simulink model "Robustness"  (R2022a)
settings: Solver=VariableStepAuto  StartTime=0.0  StopTime=10.0  RelTol=1e-3
InitFcn:
  | % NOTE: If using VoltPAQ-X1, make sure both Gain switches are set to 3.
  | K_AMP = 3;
  | % Maximum Output Voltage (V): YAW limited to 15 V. PITCH limited to 24 V.
  | VMAX_AMP_P = 24;
  | VMAX_AMP_Y = 15;
  | % Initial Angle of Pitch (rad)
  | theta_0 = -40.5*pi/180;
  | 
  | g = 9.81;
  | 
  | % Pitch and Yaw Motor Armature Resistance (Ohm)
  | R_m_p = 0.83;
  | R_m_y = 1.60;
  | 
  | % Pitch and Yaw Motor Current-Torque Constant (N.m/A)
  | K_t_p = 0.0182;
  | K_t_y = 0.0109;
  | 
  | % Pitch and Yaw Motor Voltage-Torque Constant (N.m/V)
  | K_yp = K_t_p / R_m_p;
  | K_py = K_t_y / R_m_y;
  | 
  | % Pitch and Yaw Viscous Damping Constant (N.m.s/rad)
  | B_p = 0.8;  % tuned while running simulation and experiment in parallel
  | B_y = 0.318; % identified as described in manual
  | 
  | % Mass of the Helicopter (kg)
  | m_heli = 1.3872;
  | 
  | % Mass of the Helicopter with Yoke (kg)
  | m_heli_case = 1.421;
  | 
  | % Distance from Pitch Pivot to Pitch/Front Motor and Yaw/Back Motor(m)
  | r_p = 7.75*0.0254;
  | r_y = (6+5/8)*0.0254;
  | 
  | % Pitch and Yaw Propeller Force-Thrust Constant found Experimentally (N/V)
  | K_f_p = 5*0.2074;
  | K_f_y = 3*0.1426;
  | 
  | % Pitch and Yaw Propeller Torque-Thrust Constant found Experimentally (N.m/V)
  | K_pp = K_f_p * r_p;
  | K_yy = K_f_y * r_y;
  | 
  | % Mass of Pitch/Front Motor and Yaw/Back Motor (kg)
  | m_motor_p = 0.292;
  | m_motor_y = 0.128;
  | 
  | % Mass of Pitch/Front and Yaw/Back Guard + Propeller(kg)
  | m_shield = 0.143 + 0.024;
  | 
  | % Total Mass of Pitch and Yaw Motor/Shield Assemblies (kg)
  | m_props = ( m_motor_p + m_motor_y + 2 * m_shield );
  | 
  | % Mass of Helicopter Body moving about Pitch Axis (kg)
  | m_body_p = m_heli - m_props;
  | 
  | % Mass of Helicopter Body moving about Yaw Axis (kg)
  | m_body_y = m_heli_case - m_props;
  | 
  | % Mass of Metal Shaft Moving about Yaw Axis (kg)
  | m_shaft = 0.151;
  | 
  | % Total Length of Helicopter Body (m)
  | L_body = 19*0.0254;
  | 
  | % Helicopter Center of Mass from Pivot along Pitch Axis (m)
  | l_cm = ( (m_motor_p + m_shield ) * r_p +  (m_motor_y + m_shield ) * r_y ) / ( m_props ) ;
  | 
  | % Length of Metal Shaft Moving about Yaw Axis through slip ring (m)
  | L_shaft = 11 * 0.0254;
  | 
  | % Pitch and Yaw Motor Rotor Moment of Inertia (kg.m^2)
  | J_m_p = 1.91e-6; %1.7070e-5;
  | J_m_y = 1.374e-4; %1.4471e-5;
  | 
  | % Moment of Inertia of Helicopter Body about its CM (kg.m^2)
  | J_body_p = m_body_p * L_body^2 / 12;
  | J_body_y = m_body_y * L_body^2 / 12;
  | 
  | % Moment of Inertia of Metal Shaft about Yaw Axis (kg.m^2)
  | J_shaft = m_shaft * L_shaft^2 / 3; %;0.0851;
  | 
  | % Moment of Inertia of Pitch Motor + Guard Assembly about Pivot (kg.m^2)
  | J_p = ( m_motor_p + m_shield ) * r_p^2;
  | 
  | % Moment of Inertia of Yaw Motor + Guard Assembly about Pivot (kg.m^2)
  | J_y = ( m_motor_y + m_shield ) * r_y^2;
  | 
  | % Equivalent Moment of Inertia about Pitch and Yaw Axis (kg.m^2)
  | J_eq_p = J_m_p + J_body_p + J_p + J_y;
  | J_eq_y = J_m_y + J_body_y + J_p + J_y + J_shaft;
  | 
  | 
  | %BESSEL wn=4
  | Kbes=[     68.5119  -25.1203    5.3421   -3.6881
  |    63.1652  188.4894    0.7783   19.4789];
  | 
  | xd=-20;
settings Model: Creator=rezan  LastModifiedBy=rezan

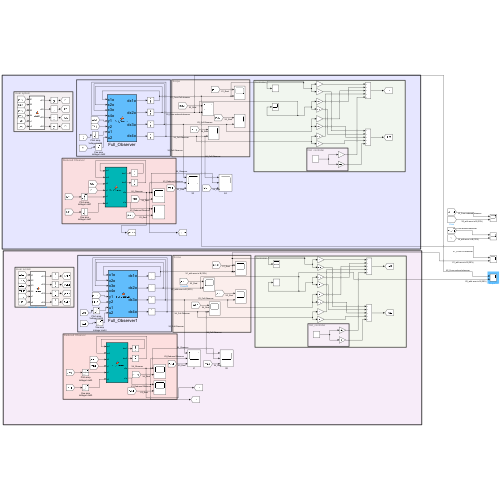
[thumbnail: Simulink's stored preview of the top-level diagram]
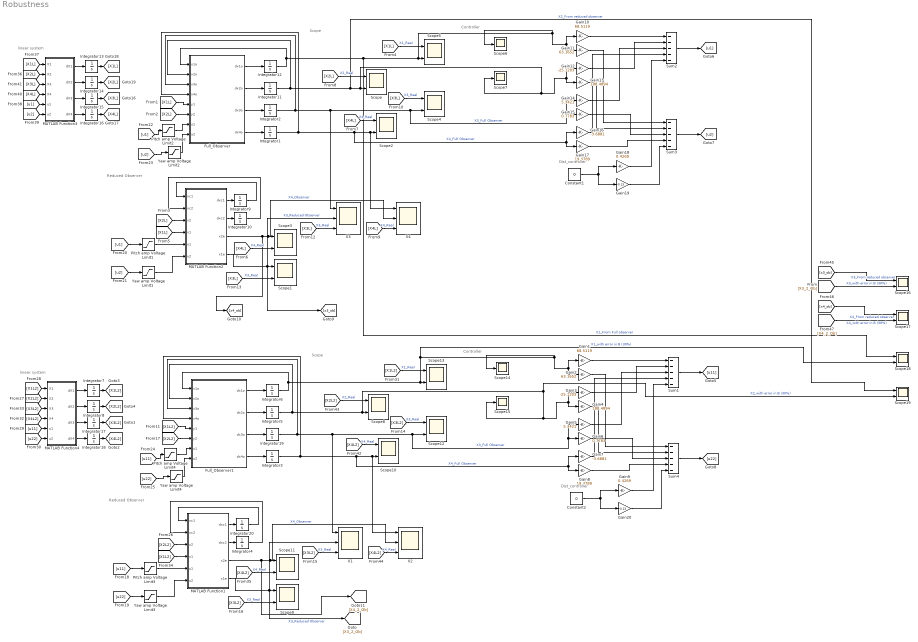
== system Robustness ==
  note: linear system
  note: Scope
  note: Reduced Observer
  note: Dist_controller
  note: Controller
  note: linear system
  note: Scope
  note: Reduced Observer
  note: Dist_controller
  note: Controller
  Constant1 : Constant  Value=0
  Constant2 : Constant  Value=0
  Full_Observer : MATLAB Function  TreatAsAtomicUnit=on
  Full_Observer1 : MATLAB Function  TreatAsAtomicUnit=on
  Gain1 : Gain  Gain=68.5119
  Gain10 : Gain  Gain=68.5119
  Gain11 : Gain  Gain=63.1652
  Gain12 : Gain  Gain=-25.1203
  Gain13 : Gain  Gain=188.4894
  Gain14 : Gain  Gain=5.3421
  Gain15 : Gain  Gain=0.7783
  Gain16 : Gain  Gain=-3.6881
  Gain17 : Gain  Gain=19.4789
  Gain18 : Gain  Gain=0.4269
  Gain19 : Gain  Gain=-0.13
  Gain2 : Gain  Gain=63.1652
  Gain20 : Gain  Gain=-0.13
  Gain3 : Gain  Gain=-25.1203
  Gain4 : Gain  Gain=188.4894
  Gain5 : Gain  Gain=5.3421
  Gain6 : Gain  Gain=0.7783
  Gain7 : Gain  Gain=-3.6881
  Gain8 : Gain  Gain=19.4789
  Gain9 : Gain  Gain=0.4269
  Integrator{1..6,8..12,14,16,18..20} (16 alike) : Integrator
  Integrator13 : Integrator  UpperSaturationLimit=40.5*pi/180  LowerSaturationLimit=-40.5*pi/180
  Integrator15 : Integrator  InitialCondition=5
  Integrator17 : Integrator  InitialCondition=5
  Integrator7 : Integrator  UpperSaturationLimit=40.5*pi/180  LowerSaturationLimit=-40.5*pi/180
  MATLAB Function1 : MATLAB Function  TreatAsAtomicUnit=on
  MATLAB Function2 : MATLAB Function  TreatAsAtomicUnit=on
  MATLAB Function3 : MATLAB Function  TreatAsAtomicUnit=on
  MATLAB Function4 : MATLAB Function  TreatAsAtomicUnit=on
  Pitch amp Voltage Limit{1..4} (4 alike) : Saturate  UpperLimit=VMAX_AMP_P  LowerLimit=- VMAX_AMP_P
  Scope{,1..5,8..13,16..19} (16 alike) : Scope  NumInputPorts=2
  Scope{6..7,14..15} (4 alike) : Scope
  Sum{1..4} (4 alike) : Sum  Inputs=-----
  X{1..4} (4 alike) : Scope  NumInputPorts=3
  Yaw amp Voltage Limit{1..4} (4 alike) : Saturate  UpperLimit=VMAX_AMP_Y  LowerLimit=- VMAX_AMP_Y
  wires:
  [X4L] -> MATLAB Function3/4(X4)
  Integrator14/1 -> [X2L]
  MATLAB Function3/1(dX1) -> Integrator13/1
  [X3L] -> MATLAB Function3/3(X3)
  MATLAB Function3/4(dX4) -> Integrator16/1
  [u1] -> MATLAB Function3/5(u1)
  [X1L] -> MATLAB Function3/1(X1)
  Integrator13/1 -> [X1L]
  MATLAB Function3/2(dX2) -> Integrator14/1
  [X2L] -> MATLAB Function3/2(X2)
  Integrator16/1 -> [X4L]
  MATLAB Function3/3(dX3) -> Integrator15/1
  [u2] -> MATLAB Function3/6(u2)
  Integrator15/1 -> [X3L]
  Gain17/1 -> Sum3/4
  Gain16/1 -> Sum2/4
  Gain13/1 -> Sum3/2
  Gain11/1 -> Sum3/1
  Sum2/1 -> [u1]
  Full_Observer/3(dx3o) -> Integrator2/1
  Gain19/1 -> Sum3/5
  Gain12/1 -> Sum2/2
  Gain15/1 -> Sum3/3
  Gain10/1 -> Sum2/1
  Sum3/1 -> [u2]
  Full_Observer/4(dx4o) -> Integrator1/1
  [X3L] -> X3/3  "X3_Real"
  [X1L] -> Scope5/1  "X1_Real"
  Constant1/1 -> Gain18/1, Gain19/1
  Yaw amp Voltage Limit2/1 -> Full_Observer/8(u2)
  Integrator10/1 -> MATLAB Function2/2(xc2)
  [X3L] -> Scope4/1  "X3_Real"
  [X4L] -> X4/3  "X4_Real"
  Integrator2/1 -> X3/1, Gain14/1, Gain15/1, Scope4/2, Full_Observer/3(x3o)  "X3_Full Observer"
  [X4L] -> Scope2/1  "X4_Real"
  Gain18/1 -> Sum2/5
  Integrator1/1 -> Gain16/1, Gain17/1, X4/1, Scope2/2, Full_Observer/4(x4o)  "X4_Full Observer"
  [X1L] -> Full_Observer/5(y1)
  Full_Observer/2(dx2o) -> Integrator11/1
  MATLAB Function2/4(x1e) -> [x3_ob], X3/2, Scope1/1  "X3_Reduced Observer"
  Gain14/1 -> Sum2/3
  [u1] -> Pitch amp Voltage Limit2/1
  [X2L] -> Scope/1  "X2_Real"
  [u2] -> Yaw amp Voltage Limit2/1
  Pitch amp Voltage Limit2/1 -> Full_Observer/7(u1)
  Integrator9/1 -> MATLAB Function2/1(xc1)
  [X2L] -> MATLAB Function2/3(x2)
  Full_Observer/1(dx1o) -> Integrator12/1
  MATLAB Function2/3(x2e) -> [x4_ob], X4/2, Scope3/1  "X4_Observer"
  [u2] -> Yaw amp Voltage Limit1/1
  MATLAB Function2/2(dxc2) -> Integrator10/1
  [X4L] -> Scope3/2  "X4_Real"
  [X2L] -> Full_Observer/6(y2)
  [X1L] -> MATLAB Function2/4(x1)
  [X3L] -> Scope1/2  "X3_Real"
  Yaw amp Voltage Limit1/1 -> MATLAB Function2/6(u2)
  Pitch amp Voltage Limit1/1 -> MATLAB Function2/5(u1)
  MATLAB Function2/1(dxc1) -> Integrator9/1
  [u1] -> Pitch amp Voltage Limit1/1
  [u11] -> Pitch amp Voltage Limit3/1
  MATLAB Function1/1(dxc1) -> Integrator20/1
  Pitch amp Voltage Limit3/1 -> MATLAB Function1/5(u1)
  Yaw amp Voltage Limit3/1 -> MATLAB Function1/6(u2)
  [X3L2] -> Scope9/2  "X3_Real"
  [X1L2] -> MATLAB Function1/4(x1)
  [X2L2] -> Full_Observer1/6(y2)
  [X4L2] -> Scope11/2  "X4_Real"
  MATLAB Function1/2(dxc2) -> Integrator4/1
  [u22] -> Yaw amp Voltage Limit3/1
  MATLAB Function1/3(x2e) -> [X4_2_Ob], Scope11/1, X2/2  "X4_Observer"
  Full_Observer1/1(dx1o) -> Integrator6/1
  Integrator5/1 -> Full_Observer1/2(x2o), Scope8/2, Scope15/1, Gain3/1, Gain4/1, Scope19/2  "X2_with error in B (30%)"
  [X2L2] -> MATLAB Function1/3(x2)
  Integrator20/1 -> MATLAB Function1/1(xc1)
  Pitch amp Voltage Limit4/1 -> Full_Observer1/7(u1)
  [u22] -> Yaw amp Voltage Limit4/1
  [X2L2] -> Scope8/1  "X2_Real"
  [u11] -> Pitch amp Voltage Limit4/1
  Gain5/1 -> Sum1/3
  MATLAB Function1/4(x1e) -> [X3_2_Ob], Scope9/1, X1/2  "X3_Reduced Observer"
  Full_Observer1/2(dx2o) -> Integrator5/1
  Integrator6/1 -> Full_Observer1/1(x1o), Scope14/1, Gain2/1, Gain1/1, Scope18/2, Scope13/2  "X1_with error in B (30%)"
  [X1L2] -> Full_Observer1/5(y1)
  Integrator3/1 -> Full_Observer1/4(x4o), Scope10/2, X2/1, Gain8/1, Gain7/1  "X4_Full Observer"
  Gain9/1 -> Sum1/5
  [X4L2] -> Scope10/1  "X4_Real"
  Integrator19/1 -> Full_Observer1/3(x3o), Scope12/2, Gain6/1, Gain5/1, X1/1  "X3_Full Observer"
  [X4L2] -> X2/3  "X4_Real"
  [X3L2] -> Scope12/1  "X3_Real"
  Integrator4/1 -> MATLAB Function1/2(xc2)
  Yaw amp Voltage Limit4/1 -> Full_Observer1/8(u2)
  Constant2/1 -> Gain20/1, Gain9/1
  [X1L2] -> Scope13/1  "X1_Real"
  [X3L2] -> X1/3  "X3_Real"
  Full_Observer1/4(dx4o) -> Integrator3/1
  Sum4/1 -> [u22]
  Gain1/1 -> Sum1/1
  Gain6/1 -> Sum4/3
  Gain3/1 -> Sum1/2
  Gain20/1 -> Sum4/5
  Full_Observer1/3(dx3o) -> Integrator19/1
  Sum1/1 -> [u11]
  Gain2/1 -> Sum4/1
  Gain4/1 -> Sum4/2
  Gain7/1 -> Sum1/4
  Gain8/1 -> Sum4/4
  Integrator17/1 -> [X3L2]
  [u22] -> MATLAB Function4/6(u2)
  MATLAB Function4/3(dX3) -> Integrator17/1
  Integrator18/1 -> [X4L2]
  [X2L2] -> MATLAB Function4/2(X2)
  MATLAB Function4/2(dX2) -> Integrator8/1
  Integrator7/1 -> [X1L2]
  [X1L2] -> MATLAB Function4/1(X1)
  [u11] -> MATLAB Function4/5(u1)
  MATLAB Function4/4(dX4) -> Integrator18/1
  [X3L2] -> MATLAB Function4/3(X3)
  MATLAB Function4/1(dX1) -> Integrator7/1
  Integrator8/1 -> [X2L2]
  [X4L2] -> MATLAB Function4/4(X4)
  [X3_2_Ob] -> Scope16/2  "X3_with error in B (30%)"
  [x3_ob] -> Scope16/1  "X3_From reduced observer"
  [x4_ob] -> Scope17/1  "X4_From reduced observer"
  [X4_2_Ob] -> Scope17/2  "X4_with error in B (30%)"
  Integrator11/1 -> Scope19/1, Gain13/1, Gain12/1, Scope7/1, Scope/2, Full_Observer/2(x2o)  "X2_From reduced observer"
  Integrator12/1 -> Gain10/1, Gain11/1, Scope6/1, Scope5/2, Scope18/1, Full_Observer/1(x1o)  "X1_From Full observer"

== matlab function Robustness/Full_Observer1 ==
  data: x1o input; dx1o output; x2o input; x3o input; x4o input; dx2o output; dx3o output; dx4o output; y1 input; y2 input; u1 input; u2 input
function [dx1o,dx2o,dx3o,dx4o] = Full_Observer(x1o,x2o,x3o,x4o,y1,y2,u1,u2)

Ao=[      0         0    1.0000         0
         0         0         0    1.0000
         0         0   -9.2751         0
         0         0         0   -3.4955];
     
Bo=[      0         0
         0         0
    2.3667    0.0790
    0.2410    0.7913];
C=[  1     0     0     0
     0     1     0     0];
u=[u1,u2].';
 
p = [-50 -50 -60 -60];
Lo = 1.0e+03 *[  0.1007         0
         0    0.1065
    2.0658         0
         0    2.6277];

xo = [x1o;x2o;x3o;x4o];
yo = C*xo;
y = [y1;y2];
dxo = Ao*xo+Bo*u+Lo*(y-yo);
dx1o = dxo(1);
dx2o = dxo(2);
dx3o = dxo(3);
dx4o = dxo(4);

== matlab function Robustness/MATLAB Function2 ==
  data: xc1 input; xc2 input; x2 input; x1 input; u1 input; dxc1 output; dxc2 output; x2e output; x1e output; u2 input
function [dxc1,dxc2,x2e,x1e] = Re_Observer(xc1,xc2,x2,x1,u1,u2)

A=[      0         0    1.0000         0
         0         0         0    1.0000
         0         0   -9.2751         0
         0         0         0   -3.4955];
     
B=[      0         0
         0         0
    2.3667    0.0790
    0.2410    0.7913];
C=[  1     0     0     0
     0     1     0     0];

 D=[  0     0
     0     0];

 
C = eye(2,4);
Aee = A(3:4,3:4);
Aes = A(3:4,1:2);
Ase = A(1:2,3:4);
Ass = A(1:2,1:2);

Be = B(3:4,1);
Bs = B(1:2,1);
u=[u1 u2];
Cs = C(1:2,1:2);
L = [   40.7249         0
         0   56.5045];

xc = [xc1;xc2];
y = [x1;x2];
xs = [x1;x2];
dxc = (Aee-L*Cs*Ase)*(xc+L*y)+(Aes*inv(Cs)-L*Cs*Ass*inv(Cs))*y+(Be-L*Cs*Bs)*u;
dxc1 = dxc(1);
dxc2 = dxc(2);
Xe = xc+L*y;
x1e = Xe(1);
x2e = Xe(2);

== matlab function Robustness/MATLAB Function3 ==
  data: X1 input; dX1 output; X2 input; X3 input; X4 input; u1 input; dX2 output; dX3 output; dX4 output; u2 input
function [dX1,dX2,dX3,dX4] = Linear(X1,X2,X3,X4,u1,u2)
%#codegen

A=[      0         0    1.0000         0
         0         0         0    1.0000
         0         0   -9.2751         0
         0         0         0   -3.4955];
     
B=[      0         0
         0         0
    2.3667    0.0790
    0.2410    0.7913];

X = [X1;X2;X3;X4];
U=[u1,u2].';
dX = A*X+B*U;
xd=0;

dX1 = dX(1);
dX2 = dX(2);
dX3 = dX(3)+xd;
dX4 = dX(4);

== matlab function Robustness/MATLAB Function1 ==
  data: xc1 input; xc2 input; x2 input; x1 input; u1 input; dxc1 output; dxc2 output; x2e output; x1e output; u2 input
function [dxc1,dxc2,x2e,x1e] = Re_Observer(xc1,xc2,x2,x1,u1,u2)

A=[      0         0    1.0000         0
         0         0         0    1.0000
         0         0   -9.2751         0
         0         0         0   -3.4955];
     
B=[      0         0
         0         0
    2.3667    0.0790
    0.2410    0.7913];
C=[  1     0     0     0
     0     1     0     0];

 D=[  0     0
     0     0];

 
C = eye(2,4);
Aee = A(3:4,3:4);
Aes = A(3:4,1:2);
Ase = A(1:2,3:4);
Ass = A(1:2,1:2);

Be = B(3:4,1);
Bs = B(1:2,1);
u=[u1 u2];
Cs = C(1:2,1:2);
L = [   40.7249         0
         0   56.5045];

xc = [xc1;xc2];
y = [x1;x2];
xs = [x1;x2];
dxc = (Aee-L*Cs*Ase)*(xc+L*y)+(Aes*inv(Cs)-L*Cs*Ass*inv(Cs))*y+(Be-L*Cs*Bs)*u;
dxc1 = dxc(1);
dxc2 = dxc(2);
Xe = xc+L*y;
x1e = Xe(1);
x2e = Xe(2);

== matlab function Robustness/MATLAB Function4 ==
  data: X1 input; dX1 output; X2 input; X3 input; X4 input; u1 input; dX2 output; dX3 output; dX4 output; u2 input
function [dX1,dX2,dX3,dX4] = Linear(X1,X2,X3,X4,u1,u2)
%#codegen

A=[      0         0    1.0000         0
         0         0         0    1.0000
         0         0   -9.2751         0
         0         0         0   -3.4955];
     
B=[      0         0
         0         0
    2.3667    0.0790
    0.2410    0.7913];

X = [X1;X2;X3;X4];
U=[u1,u2].';
B=0.3*B+B;
dX = A*X+B*U;
xd=0;

dX1 = dX(1);
dX2 = dX(2);
dX3 = dX(3)+xd;
dX4 = dX(4);

== matlab function Robustness/Full_Observer ==
  data: x1o input; dx1o output; x2o input; x3o input; x4o input; dx2o output; dx3o output; dx4o output; y1 input; y2 input; u1 input; u2 input
function [dx1o,dx2o,dx3o,dx4o] = Full_Observer(x1o,x2o,x3o,x4o,y1,y2,u1,u2)

Ao=[      0         0    1.0000         0
         0         0         0    1.0000
         0         0   -9.2751         0
         0         0         0   -3.4955];
     
Bo=[      0         0
         0         0
    2.3667    0.0790
    0.2410    0.7913];
C=[  1     0     0     0
     0     1     0     0];
u=[u1,u2].';
 
p = [-50 -50 -60 -60];
Lo = 1.0e+03 *[  0.1007         0
         0    0.1065
    2.0658         0
         0    2.6277];

xo = [x1o;x2o;x3o;x4o];
yo = C*xo;
y = [y1;y2];
dxo = Ao*xo+Bo*u+Lo*(y-yo);
dx1o = dxo(1);
dx2o = dxo(2);
dx3o = dxo(3);
dx4o = dxo(4);
